simulink subsystem "car_complex_simulink"  (R2025b)
settings: Solver=VariableStepAuto  StartTime=0.0  StopTime=10.0  RelTol=1e-3
settings Model: Creator=sanborkl  LastModifiedBy=sanborkl

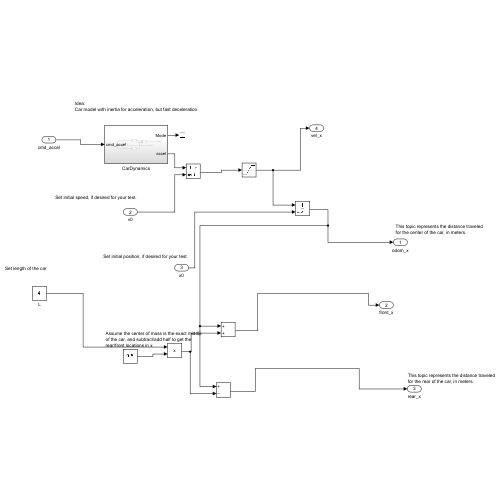
[thumbnail: Simulink's stored preview of the top-level diagram]
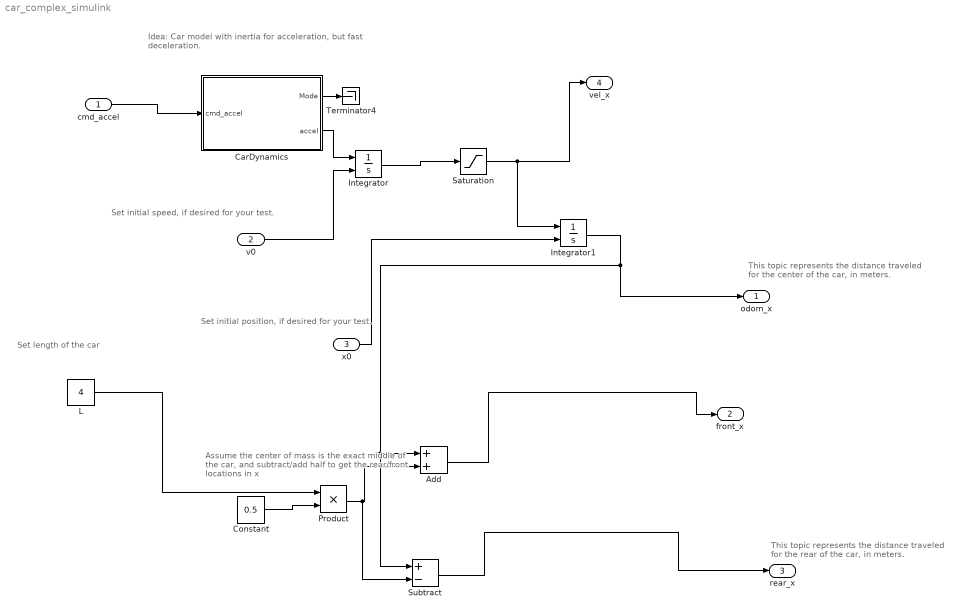
== system car_complex_simulink ==
  note: Assume the center of mass is the exact middle
      | of the car, and subtract/add half to get the
      | rear/front locations in x
  note: Set length of the car
  note: Set initial speed, if desired for your test.
  note: Set initial position, if desired for your test.
  note: Idea:
      | Car model with inertia for acceleration, but fast deceleration.
  note: This topic represents the distance traveled
      | for the rear of the car, in meters.
  note: This topic represents the distance traveled
      | for the center of the car, in meters.
  cmd_accel : Inport
  v0 : Inport  Port=2
  x0 : Inport  Port=3
  Add : Sum
  CarDynamics : Subsystem
  Constant : Constant  Value=0.5
  Integrator : Integrator  InitialConditionSource=external  LimitOutput=on  UpperSaturationLimit=40  LowerSaturationLimit=0
  Integrator1 : Integrator  InitialConditionSource=external
  L : Constant  Value=4
  Product : Product
  Saturation : Saturate  UpperLimit=40  LowerLimit=0
  Subtract : Sum  Inputs=+-
  Terminator4 : Terminator
  odom_x : Outport
  front_x : Outport  Port=2
  rear_x : Outport  Port=3
  vel_x : Outport  Port=4
  wires:
  Subtract/1 -> rear_x/1
  x0/1 -> Integrator1/2
  CarDynamics/1(Mode) -> Terminator4/1
  CarDynamics/2(accel) -> Integrator/1
  Saturation/1 -> vel_x/1, Integrator1/1
  Integrator1/1 -> odom_x/1, Subtract/1, Add/1
  v0/1 -> Integrator/2
  Add/1 -> front_x/1
  Product/1 -> Subtract/2, Add/2
  Constant/1 -> Product/2
  Integrator/1 -> Saturation/1
  L/1 -> Product/1
  cmd_accel/1 -> CarDynamics/1(cmd_accel)

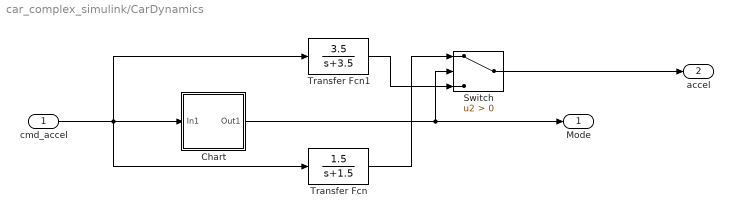
== system car_complex_simulink/CarDynamics ==
  cmd_accel : Inport
  Chart : Stateflow chart  TreatAsAtomicUnit=on
  Switch : Switch  Criteria=u2 > Threshold  SaturateOnIntegerOverflow=off  InputSameDT=off
  Transfer Fcn : TransferFcn  Numerator=[1.5]  Denominator=[1 1.5]
  Transfer Fcn1 : TransferFcn  Numerator=[3.5]  Denominator=[1 3.5]
  Mode : Outport
  accel : Outport  Port=2
  wires:
  cmd_accel/1 -> Chart/1(In1), Transfer Fcn/1, Transfer Fcn1/1
  Transfer Fcn1/1 -> Switch/3
  Switch/1 -> accel/1
  Transfer Fcn/1 -> Switch/1
  Chart/1(Out1) -> Mode/1, Switch/2

== stateflow chart car_complex_simulink/CarDynamics/Chart ==
  state Default
    entry: Out1=1;
  state Slowing
    entry: Out1=-1;
  (default) -> Default
  Slowing -> Default : [In1 > 0]
  Default -> Slowing : [In1 < 0.2]
  data: In1 input; Out1 output
